simulink model "PEP3"  (R2024b)
settings: Solver=VariableStepAuto  StartTime=0.0  StopTime=0.1  RelTol=1e-6
values from neighbouring files (symbols this model uses):
  f = 1500    [P4.m]    (also in Proiect3_1.m; ProiectEP_3.m; ProiectEP_Init.m; Proiect_2.m)
  Hc = (1/Hf) * (H0/(1-H0))    [Proiect3_1.m]    (also in ProiectEP_3.m = minreal( inv(Hp) * (Ho/(1 - Ho)) ))
undefined symbols (not defined in the file or in its folder): den, num
settings Model: DataDictionary=SampleTime.sldd  Creator=Razvan  LastModifiedBy=Razvan

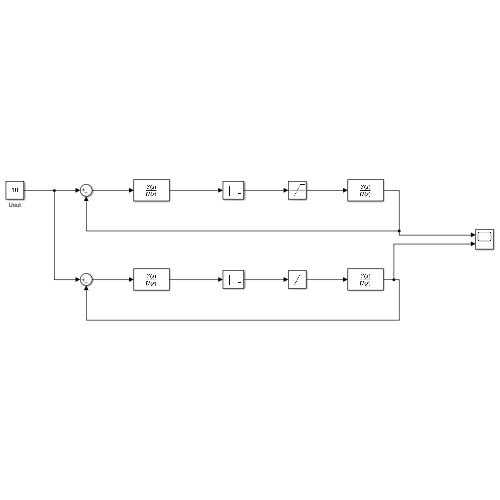
[thumbnail: Simulink's stored preview of the top-level diagram]
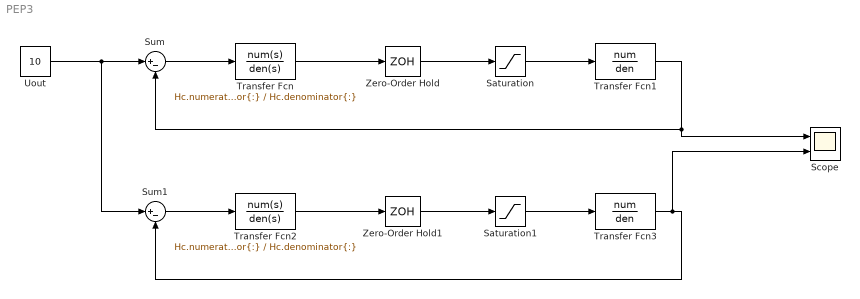
== system PEP3 ==
  Saturation : Saturate  UpperLimit=1  LowerLimit=0
  Saturation1 : Saturate  UpperLimit=1  LowerLimit=0
  Scope : Scope  NumInputPorts=2
  Sum : Sum  Inputs=|+-
  Sum1 : Sum  Inputs=|+-
  Transfer Fcn : TransferFcn  Numerator=Hc.numerator{:}  Denominator=Hc.denominator{:}
  Transfer Fcn1 : TransferFcn  Numerator=num  Denominator=den
  Transfer Fcn2 : TransferFcn  Numerator=Hc.numerator{:}  Denominator=Hc.denominator{:}
  Transfer Fcn3 : TransferFcn  Numerator=num  Denominator=den
  Uout : Constant  Value=10
  Zero-Order Hold : ZeroOrderHold  SampleTime=1/f/10
  Zero-Order Hold1 : ZeroOrderHold  SampleTime=1/f
  wires:
  Transfer Fcn/1 -> Zero-Order Hold/1
  Saturation/1 -> Transfer Fcn1/1
  Sum/1 -> Transfer Fcn/1
  Transfer Fcn1/1 -> Scope/1, Sum/2
  Uout/1 -> Sum1/1, Sum/1
  Zero-Order Hold/1 -> Saturation/1
  Transfer Fcn2/1 -> Zero-Order Hold1/1
  Saturation1/1 -> Transfer Fcn3/1
  Zero-Order Hold1/1 -> Saturation1/1
  Sum1/1 -> Transfer Fcn2/1
  Transfer Fcn3/1 -> Scope/2, Sum1/2
